simulink model "het_platoon_model"  (R2018b)
settings: Solver=ode1  StartTime=0.0  StopTime=simDrv.time_s(end)  FixedStep=sim_t_step  RelTol=1e-3
values from neighbouring files (symbols this model uses):
  sim_t_step = 0.01    [startHetPlatoonModel.m]
undefined symbols (not defined in the file or in its folder): adj_motEffMap, CTModel, DiscIntNeverNeededParam, LT, motSpdVec, motTrqVec, msk_mot_cont_trq, msk_mot_num, msk_mot_spd_bpt, MT, N_OptResults, simDrv, SPHETModel, TT
libraries: platooning_custom_blocks x24, simulink x7, dspstat3 x1, custom_func x1
(part 1 of 3)
PauseFcn:
  | runOptSPHET
settings Model: Creator=amankalia  LastModifiedBy=Aman-Home

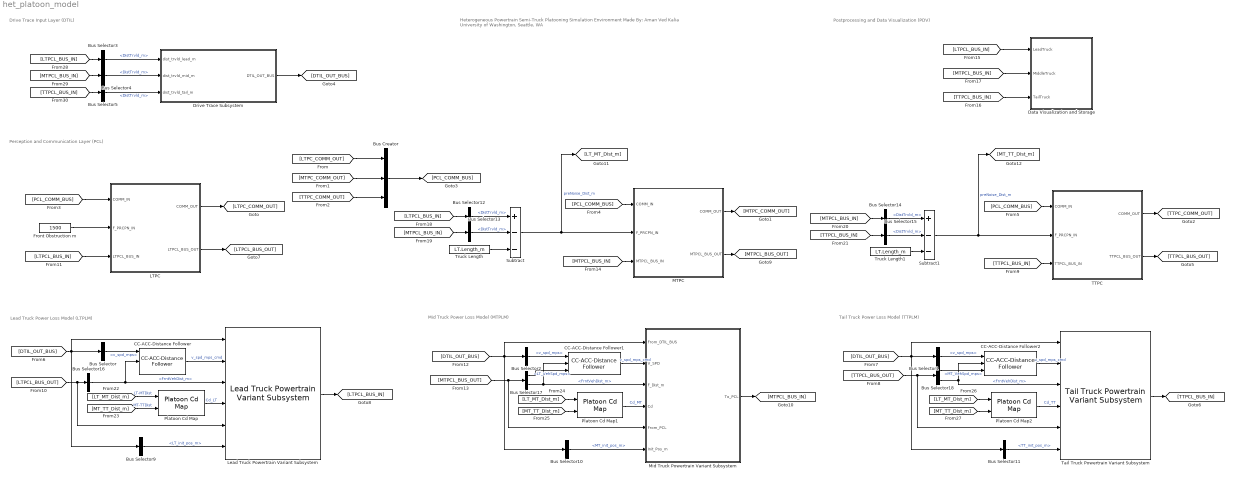
== system het_platoon_model ==
  note: Heterogeneous Powertrain Semi-Truck
      | Platooning Simulation Environment
      |
      | Made By: Aman Ved Kalia
      | University of Washington, Seattle, WA
  note: Lead Truck Power Loss Model (LTPLM)
  note: Perception and Communication Layer (PCL)
  note: Drive Trace Input Layer (DTIL)
  note: Mid Truck Power Loss Model (MTPLM)
  note: Tail Truck Power Loss Model (TTPLM)
  note: Postprocessing and Data Visualization (PDV)
  Bus Creator : BusCreator  Inputs=3
  Bus Selector : BusSelector  OutputSignals=v_spd_mps
  Bus Selector1 : BusSelector  OutputSignals=v_spd_mps
  Bus Selector10 : BusSelector  OutputSignals=MT_init_pos_m
  Bus Selector11 : BusSelector  OutputSignals=TT_init_pos_m
  Bus Selector{3..5,12..15} (7 alike) : BusSelector  OutputSignals=State_BUS.DistTrvld_m
  Bus Selector16 : BusSelector  OutputSignals=FrntVehDist_m
  Bus Selector17 : BusSelector  OutputSignals=LT_VehSpd_mps,FrntVehDist_m
  Bus Selector18 : BusSelector  OutputSignals=MT_VehSpd_mps,FrntVehDist_m
  Bus Selector2 : BusSelector  OutputSignals=v_spd_mps
  Bus Selector9 : BusSelector  OutputSignals=LT_init_pos_m
  CC-ACC-Distance Follower : platooning_custom_blocks/CC-ACC-Distance Follower  msk_cc_mode=Disabled  msk_cc_setspd=25  msk_cc_time=100  msk_ACC_Kp=0.5  msk_ACC_Ki=0.01  msk_ACC_Kd=0  msk_ACC_setdist_init=70  msk_platoon_time=200  msk_ACC_setdist_final=15
  CC-ACC-Distance Follower1 : platooning_custom_blocks/CC-ACC-Distance Follower  msk_cc_mode=Disabled  msk_cc_setspd=28  msk_cc_time=100  msk_ACC_Kp=1  msk_ACC_Ki=0.05  msk_ACC_Kd=0.01  msk_ACC_setdist_init=60  msk_platoon_time=200  msk_ACC_setdist_final=40
  CC-ACC-Distance Follower2 : platooning_custom_blocks/CC-ACC-Distance Follower  msk_cc_mode=Disabled  msk_cc_setspd=28  msk_cc_time=100  msk_ACC_Kp=1  msk_ACC_Ki=0.05  msk_ACC_Kd=0.01  msk_ACC_setdist_init=60  msk_platoon_time=200  msk_ACC_setdist_final=40
  Data Visualization and Storage : Subsystem
  Drive Trace Subsystem : Subsystem
  Front Obstruction m : Constant  Value=1500
  LTPC : Subsystem
  Lead Truck Powertrain Variant Subsystem : platooning_custom_blocks/Lead Truck Powertrain Variant Subsystem  SystemSampleTime=-1
  MTPC : Subsystem
  Mid Truck Powertrain Variant Subsystem : Subsystem  AncestorBlock=platooning_custom_blocks/Mid Truck Powertrain Variant Subsystem  Variant=on
  Platoon Cd Map : platooning_custom_blocks/Platoon Cd Map  msk_platoon_type=Individual  pos=Lead  msk_platoon_cd_map=Cd_Map  msk_platoon_cd_map_t2=Cd_Map_T2  msk_d1_bpt=d_11  msk_d2_bpt=d_22  msk_cd_avg=0.52
  Platoon Cd Map1 : platooning_custom_blocks/Platoon Cd Map  msk_platoon_type=Individual  pos=Middle  msk_platoon_cd_map=Cd_Map  msk_platoon_cd_map_t2=Cd_Map_T2  msk_d1_bpt=d_11  msk_d2_bpt=d_22  msk_cd_avg=0.52
  Platoon Cd Map2 : platooning_custom_blocks/Platoon Cd Map  msk_platoon_type=Individual  pos=Tail  msk_platoon_cd_map=Cd_Map  msk_platoon_cd_map_t2=Cd_Map_T2  msk_d1_bpt=d_11  msk_d2_bpt=d_22  msk_cd_avg=0.52
  Subtract : Sum  Inputs=+--
  Subtract1 : Sum  Inputs=+--
  TTPC : Subsystem
  Tail Truck Powertrain Variant Subsystem : platooning_custom_blocks/Tail Truck Powertrain Variant Subsystem  SystemSampleTime=-1
  Truck Length : Constant  Value=LT.Length_m
  Truck Length1 : Constant  Value=LT.Length_m
  wires:
  Drive Trace Subsystem/1(DTIL_OUT_BUS) -> [DTIL_OUT_BUS]
  LTPC/1(COMM_OUT) -> [LTPC_COMM_OUT]
  MTPC/1(COMM_OUT) -> [MTPC_COMM_OUT]
  TTPC/1(COMM_OUT) -> [TTPC_COMM_OUT]
  [LTPC_COMM_OUT] -> Bus Creator/1
  [MTPC_COMM_OUT] -> Bus Creator/2
  [TTPC_COMM_OUT] -> Bus Creator/3
  Bus Creator/1 -> [PCL_COMM_BUS]
  Bus Selector16/1 -> Lead Truck Powertrain Variant Subsystem/3, CC-ACC-Distance Follower/2  "<FrntVehDist_m>"
  Bus Selector/1 -> CC-ACC-Distance Follower/1  "<v_spd_mps>"
  [DTIL_OUT_BUS] -> Bus Selector/1, Lead Truck Powertrain Variant Subsystem/1, Bus Selector9/1
  CC-ACC-Distance Follower/1 -> Lead Truck Powertrain Variant Subsystem/2  "v_spd_mps_cmd"
  Bus Selector18/2 -> Tail Truck Powertrain Variant Subsystem/3, CC-ACC-Distance Follower2/2  "<FrntVehDist_m>"
  [DTIL_OUT_BUS] -> Bus Selector11/1, Bus Selector1/1, Tail Truck Powertrain Variant Subsystem/1
  Bus Selector1/1 -> CC-ACC-Distance Follower2/1  "<v_spd_mps>"
  CC-ACC-Distance Follower2/1 -> Tail Truck Powertrain Variant Subsystem/2  "v_spd_mps_cmd"
  TTPC/2(TTPCL_BUS_OUT) -> [TTPCL_BUS_OUT]
  [TTPCL_BUS_OUT] -> Tail Truck Powertrain Variant Subsystem/5, Bus Selector18/1
  Tail Truck Powertrain Variant Subsystem/1 -> [TTPCL_BUS_IN]
  [TTPCL_BUS_IN] -> TTPC/3(TTPCL_BUS_IN)
  LTPC/2(LTPCL_BUS_OUT) -> [LTPCL_BUS_OUT]
  [LTPCL_BUS_OUT] -> Bus Selector16/1, Lead Truck Powertrain Variant Subsystem/5
  Lead Truck Powertrain Variant Subsystem/1 -> [LTPCL_BUS_IN]
  [LTPCL_BUS_IN] -> LTPC/3(LTPCL_BUS_IN)
  [DTIL_OUT_BUS] -> Bus Selector10/1, Mid Truck Powertrain Variant Subsystem/1(From_DTIL_BUS), Bus Selector2/1
  CC-ACC-Distance Follower1/1 -> Mid Truck Powertrain Variant Subsystem/2(V_SPD)  "v_spd_mps_cmd"
  Bus Selector17/2 -> Mid Truck Powertrain Variant Subsystem/3(F_Dist_m), CC-ACC-Distance Follower1/2  "<FrntVehDist_m>"
  [MTPCL_BUS_OUT] -> Mid Truck Powertrain Variant Subsystem/5(From_PCL), Bus Selector17/1
  Bus Selector2/1 -> CC-ACC-Distance Follower1/1  "<v_spd_mps>"
  Mid Truck Powertrain Variant Subsystem/1(To_PCL) -> [MTPCL_BUS_IN]
  MTPC/2(MTPCL_BUS_OUT) -> [MTPCL_BUS_OUT]
  [MTPCL_BUS_IN] -> MTPC/3(MTPCL_BUS_IN)
  [PCL_COMM_BUS] -> LTPC/1(COMM_IN)
  [PCL_COMM_BUS] -> MTPC/1(COMM_IN)
  [PCL_COMM_BUS] -> TTPC/1(COMM_IN)
  Bus Selector9/1 -> Lead Truck Powertrain Variant Subsystem/6  "<LT_init_pos_m>"
  Bus Selector10/1 -> Mid Truck Powertrain Variant Subsystem/6(Init_Pos_m)  "<MT_init_pos_m>"
  Bus Selector11/1 -> Tail Truck Powertrain Variant Subsystem/6  "<TT_init_pos_m>"
  [LTPCL_BUS_IN] -> Bus Selector12/1
  [MTPCL_BUS_IN] -> Bus Selector13/1
  Bus Selector12/1 -> Subtract/1  "<DistTrvld_m>"
  Bus Selector13/1 -> Subtract/2  "<DistTrvld_m>"
  Truck Length/1 -> Subtract/3
  Truck Length1/1 -> Subtract1/3
  Bus Selector14/1 -> Subtract1/1  "<DistTrvld_m>"
  Bus Selector15/1 -> Subtract1/2  "<DistTrvld_m>"
  [MTPCL_BUS_IN] -> Bus Selector14/1
  [TTPCL_BUS_IN] -> Bus Selector15/1
  Front Obstruction m/1 -> LTPC/2(F_PRCPN_IN)
  Bus Selector17/1 -> CC-ACC-Distance Follower1/3  "<LT_VehSpd_mps>"
  Bus Selector18/1 -> CC-ACC-Distance Follower2/3  "<MT_VehSpd_mps>"
  Platoon Cd Map/1 -> Lead Truck Powertrain Variant Subsystem/4  "Cd_LT"
  [LT_MT_Dist_m] -> Platoon Cd Map/1  "LT-MTDist"
  [MT_TT_Dist_m] -> Platoon Cd Map/2  "MT-TTDist"
  [MT_TT_Dist_m] -> Platoon Cd Map1/2
  [LT_MT_Dist_m] -> Platoon Cd Map1/1
  Platoon Cd Map1/1 -> Mid Truck Powertrain Variant Subsystem/4(Cd)  "Cd_MT"
  [MT_TT_Dist_m] -> Platoon Cd Map2/2
  [LT_MT_Dist_m] -> Platoon Cd Map2/1
  Platoon Cd Map2/1 -> Tail Truck Powertrain Variant Subsystem/4  "Cd_TT"
  Subtract1/1 -> [MT_TT_Dist_m], TTPC/2(F_PRCPN_IN)  "preNoise_Dist_m"
  Subtract/1 -> [LT_MT_Dist_m], MTPC/2(F_PRCPN_IN)  "preNoise_Dist_m"
  [LTPCL_BUS_IN] -> Data Visualization and Storage/1(LeadTruck)
  [MTPCL_BUS_IN] -> Data Visualization and Storage/2(MiddleTruck)
  [TTPCL_BUS_IN] -> Data Visualization and Storage/3(TailTruck)
  [LTPCL_BUS_IN] -> Bus Selector3/1
  Bus Selector3/1 -> Drive Trace Subsystem/1(dist_trvld_lead_m)  "<DistTrvld_m>"
  [MTPCL_BUS_IN] -> Bus Selector4/1
  Bus Selector4/1 -> Drive Trace Subsystem/2(dist_trvld_mid_m)  "<DistTrvld_m>"
  [TTPCL_BUS_IN] -> Bus Selector5/1
  Bus Selector5/1 -> Drive Trace Subsystem/3(dist_trvld_tail_m)  "<DistTrvld_m>"

== system het_platoon_model/Data Visualization and Storage ==
  LeadTruck : Inport
  MiddleTruck : Inport  Port=2
  TailTruck : Inport  Port=3
  Bus Creator : BusCreator  Inputs=3
  Bus Creator1 : BusCreator  Inputs=3
  Bus Creator2 : BusCreator  Inputs=3
  Bus Selector3 : BusSelector  OutputSignals=EC_BUS,FC_BUS,State_BUS
  Bus Selector5 : BusSelector  OutputSignals=EC_BUS,State_BUS,FC_BUS
  Bus Selector7 : BusSelector  OutputSignals=EC_BUS,FC_BUS,State_BUS
  Scope{,1..7} (8 alike) : Scope
  To Workspace : ToWorkspace  VariableName=TT_SimData  SaveFormat=Timeseries  SampleTime=-1
  To Workspace1 : ToWorkspace  VariableName=LT_SimData  SaveFormat=Timeseries  SampleTime=-1
  To Workspace2 : ToWorkspace  VariableName=MT_SimData  SaveFormat=Timeseries  SampleTime=-1
  wires:
  Bus Selector3/2 -> Bus Creator1/2, Scope1/1  "<FC_BUS>"
  Bus Selector7/3 -> Scope7/1, Bus Creator2/3  "<State_BUS>"
  Bus Selector5/1 -> Bus Creator/1, Scope3/1  "<EC_BUS>"
  Bus Selector7/1 -> Bus Creator2/1, Scope5/1  "<EC_BUS>"
  Bus Selector3/3 -> Scope2/1, Bus Creator1/3  "<State_BUS>"
  TailTruck/1 -> Bus Selector5/1
  Bus Selector5/2 -> Scope4/1, Bus Creator/2  "<State_BUS>"
  Bus Selector7/2 -> Bus Creator2/2, Scope6/1  "<FC_BUS>"
  Bus Selector3/1 -> Bus Creator1/1, Scope/1  "<EC_BUS>"
  LeadTruck/1 -> Bus Selector3/1
  MiddleTruck/1 -> Bus Selector7/1
  Bus Creator/1 -> To Workspace/1
  Bus Creator1/1 -> To Workspace1/1
  Bus Creator2/1 -> To Workspace2/1
  Bus Selector5/3 -> Bus Creator/3  "<FC_BUS>"

== system het_platoon_model/Drive Trace Subsystem ==
  note: simDrv.dist_mi * 1609.34
  note: simDrv.rand_spd_mph * 0.44704
  dist_trvld_lead_m : Inport
  dist_trvld_mid_m : Inport  Port=2
  dist_trvld_tail_m : Inport  Port=3
  Bus Creator : BusCreator  Inputs=8
  Clock : Clock
  Constant : Constant  Value=LT.Init_Pos_m
  Constant1 : Constant  Value=MT.Init_Pos_m
  Constant2 : Constant  Value=TT.Init_Pos_m
  Cycle Distance : Constant  Commented=on  Value=simDrv.dist_mi(end) * 1609.34
  Distance vs Grade LUT1 : Lookup_n-D  NumberOfTableDimensions=1  BreakpointsForDimension1=simDrv.dist_m(2:6)  Table=simDrv.grade_pct(2:6)  ExtrapMethod=Clip  UseLastTableValue=on  InternalRulePriority=Speed  RndMeth=Simplest  InputSameDT=on
  Distance vs Grade LUT2 : Lookup_n-D  NumberOfTableDimensions=1  BreakpointsForDimension1=simDrv.dist_m(2:6)  Table=simDrv.grade_pct(2:6)  ExtrapMethod=Clip  UseLastTableValue=on  InternalRulePriority=Speed  RndMeth=Simplest  InputSameDT=on
  Distance vs Grade LUT3 : Lookup_n-D  NumberOfTableDimensions=1  BreakpointsForDimension1=simDrv.dist_m(2:6)  Table=simDrv.grade_pct(2:6)  ExtrapMethod=Clip  UseLastTableValue=on  InternalRulePriority=Speed  RndMeth=Simplest  InputSameDT=on
  GreaterThan : RelationalOperator  Commented=on  OutDataTypeStr=boolean  RndMeth=Simplest
  GreaterThan1 : RelationalOperator  Commented=on  OutDataTypeStr=boolean  RndMeth=Simplest
  GreaterThan2 : RelationalOperator  Commented=on  OutDataTypeStr=boolean  RndMeth=Simplest
  Logical Operator : Logic  Commented=on  Inputs=3  AllPortsSameDT=off  OutDataTypeStr=boolean
  Speed vs Time LUT : Lookup_n-D  NumberOfTableDimensions=1  BreakpointsForDimension1=simDrv.time_s  Table=simDrv.spd_mps  ExtrapMethod=Clip  UseLastTableValue=on  InternalRulePriority=Speed  RndMeth=Simplest  InputSameDT=on
  Stop Simulation : Stop  Commented=on
  DTIL_OUT_BUS : Outport
  wires:
  dist_trvld_lead_m/1 -> GreaterThan/1, Distance vs Grade LUT1/1
  Bus Creator/1 -> DTIL_OUT_BUS/1  "DTIL_OUT_BUS"
  Distance vs Grade LUT1/1 -> Bus Creator/3  "lead_grade_pct"
  Speed vs Time LUT/1 -> Bus Creator/2  "v_spd_mps"
  Clock/1 -> Bus Creator/1, Speed vs Time LUT/1  "clock"
  dist_trvld_mid_m/1 -> GreaterThan1/1, Distance vs Grade LUT2/1
  dist_trvld_tail_m/1 -> GreaterThan2/1, Distance vs Grade LUT3/1
  Distance vs Grade LUT2/1 -> Bus Creator/4  "mid_grade_pct"
  Distance vs Grade LUT3/1 -> Bus Creator/5  "tail_grade_pct"
  Constant/1 -> Bus Creator/6  "LT_init_pos_m"
  Constant1/1 -> Bus Creator/7  "MT_init_pos_m"
  Constant2/1 -> Bus Creator/8  "TT_init_pos_m"
  Cycle Distance/1 -> GreaterThan/2, GreaterThan1/2, GreaterThan2/2
  GreaterThan1/1 -> Logical Operator/2
  GreaterThan/1 -> Logical Operator/1
  GreaterThan2/1 -> Logical Operator/3
  Logical Operator/1 -> Stop Simulation/1

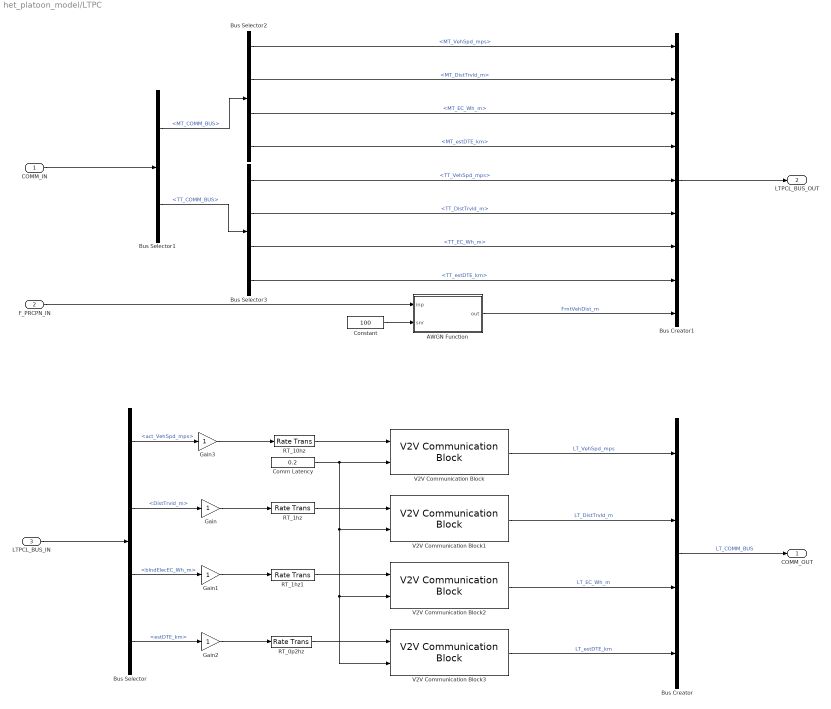
== system het_platoon_model/LTPC ==
  COMM_IN : Inport
  F_PRCPN_IN : Inport  Port=2
  LTPCL_BUS_IN : Inport  Port=3
  AWGN Function : MATLAB Function  TreatAsAtomicUnit=on
  Bus Creator : BusCreator  Inputs=4
  Bus Creator1 : BusCreator  Inputs=9
  Bus Selector : BusSelector  OutputSignals=State_BUS.act_VehSpd_mps,State_BUS.DistTrvld_m,EC_BUS.blndElecEC_Wh_m,State_BUS.estDTE_km
  Bus Selector1 : BusSelector  OutputSignals=MT_COMM_BUS,TT_COMM_BUS
  Bus Selector2 : BusSelector  OutputSignals=MT_VehSpd_mps,MT_DistTrvld_m,MT_EC_Wh_m,MT_estDTE_km
  Bus Selector3 : BusSelector  OutputSignals=TT_VehSpd_mps,TT_DistTrvld_m,TT_EC_Wh_m,TT_estDTE_km
  Comm Latency : Constant  Value=0.2
  Constant : Constant  Value=100
  Gain{,1..3} (4 alike) : Gain
  RT_0p2hz : RateTransition  OutPortSampleTime=1
  RT_10hz : RateTransition  OutPortSampleTime=0.1
  RT_1hz : RateTransition  OutPortSampleTime=1
  RT_1hz1 : RateTransition  OutPortSampleTime=1
  V2V Communication Block{,1..3} (4 alike) : platooning_custom_blocks/V2V Communication Block  msk_t_step_s=sim_t_step  msk_snr_value=100
  COMM_OUT : Outport
  LTPCL_BUS_OUT : Outport  Port=2
  wires:
  Bus Creator/1 -> COMM_OUT/1  "LT_COMM_BUS"
  Bus Creator1/1 -> LTPCL_BUS_OUT/1
  COMM_IN/1 -> Bus Selector1/1
  F_PRCPN_IN/1 -> AWGN Function/1(inp)
  LTPCL_BUS_IN/1 -> Bus Selector/1
  Bus Selector/2 -> Gain/1  "<DistTrvld_m>"
  Bus Selector/3 -> Gain1/1  "<blndElecEC_Wh_m>"
  Gain/1 -> RT_1hz/1
  Gain1/1 -> RT_1hz1/1
  Bus Selector/4 -> Gain2/1  "<estDTE_km>"
  Gain2/1 -> RT_0p2hz/1
  Constant/1 -> AWGN Function/2(snr)
  AWGN Function/1(out) -> Bus Creator1/9  "FrntVehDist_m"
  Bus Selector/1 -> Gain3/1  "<act_VehSpd_mps>"
  Gain3/1 -> RT_10hz/1
  RT_10hz/1 -> V2V Communication Block/1
  RT_1hz/1 -> V2V Communication Block1/1
  RT_1hz1/1 -> V2V Communication Block2/1
  RT_0p2hz/1 -> V2V Communication Block3/1
  V2V Communication Block3/1 -> Bus Creator/4  "LT_estDTE_km"
  V2V Communication Block2/1 -> Bus Creator/3  "LT_EC_Wh_m"
  V2V Communication Block1/1 -> Bus Creator/2  "LT_DistTrvld_m"
  V2V Communication Block/1 -> Bus Creator/1  "LT_VehSpd_mps"
  Comm Latency/1 -> V2V Communication Block3/2, V2V Communication Block2/2, V2V Communication Block1/2, V2V Communication Block/2
  Bus Selector1/1 -> Bus Selector2/1  "<MT_COMM_BUS>"
  Bus Selector1/2 -> Bus Selector3/1  "<TT_COMM_BUS>"
  Bus Selector3/4 -> Bus Creator1/8  "<TT_estDTE_km>"
  Bus Selector3/3 -> Bus Creator1/7  "<TT_EC_Wh_m>"
  Bus Selector3/2 -> Bus Creator1/6  "<TT_DistTrvld_m>"
  Bus Selector3/1 -> Bus Creator1/5  "<TT_VehSpd_mps>"
  Bus Selector2/4 -> Bus Creator1/4  "<MT_estDTE_km>"
  Bus Selector2/3 -> Bus Creator1/3  "<MT_EC_Wh_m>"
  Bus Selector2/2 -> Bus Creator1/2  "<MT_DistTrvld_m>"
  Bus Selector2/1 -> Bus Creator1/1  "<MT_VehSpd_mps>"

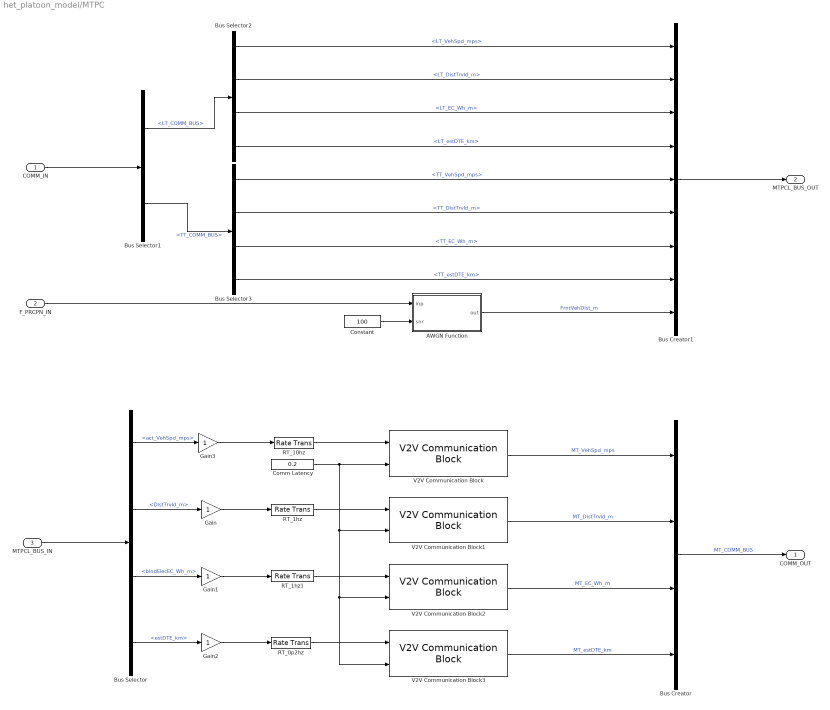
== system het_platoon_model/MTPC ==
  COMM_IN : Inport
  F_PRCPN_IN : Inport  Port=2
  MTPCL_BUS_IN : Inport  Port=3
  AWGN Function : MATLAB Function  TreatAsAtomicUnit=on
  Bus Creator : BusCreator  Inputs=4
  Bus Creator1 : BusCreator  Inputs=9
  Bus Selector : BusSelector  OutputSignals=State_BUS.act_VehSpd_mps,State_BUS.DistTrvld_m,EC_BUS.blndElecEC_Wh_m,State_BUS.estDTE_km
  Bus Selector1 : BusSelector  OutputSignals=LT_COMM_BUS,TT_COMM_BUS
  Bus Selector2 : BusSelector  OutputSignals=LT_VehSpd_mps,LT_DistTrvld_m,LT_EC_Wh_m,LT_estDTE_km
  Bus Selector3 : BusSelector  OutputSignals=TT_VehSpd_mps,TT_DistTrvld_m,TT_EC_Wh_m,TT_estDTE_km
  Comm Latency : Constant  Value=0.2
  Constant : Constant  Value=100
  Gain{,1..3} (4 alike) : Gain
  RT_0p2hz : RateTransition  OutPortSampleTime=1
  RT_10hz : RateTransition  OutPortSampleTime=0.1
  RT_1hz : RateTransition  OutPortSampleTime=1
  RT_1hz1 : RateTransition  OutPortSampleTime=1
  V2V Communication Block{,1..3} (4 alike) : platooning_custom_blocks/V2V Communication Block  msk_t_step_s=sim_t_step  msk_snr_value=100
  COMM_OUT : Outport
  MTPCL_BUS_OUT : Outport  Port=2
  wires:
  Bus Creator/1 -> COMM_OUT/1  "MT_COMM_BUS"
  Bus Creator1/1 -> MTPCL_BUS_OUT/1
  COMM_IN/1 -> Bus Selector1/1
  F_PRCPN_IN/1 -> AWGN Function/1(inp)
  MTPCL_BUS_IN/1 -> Bus Selector/1
  Bus Selector/2 -> Gain/1  "<DistTrvld_m>"
  Bus Selector/3 -> Gain1/1  "<blndElecEC_Wh_m>"
  Gain/1 -> RT_1hz/1
  Gain1/1 -> RT_1hz1/1
  Bus Selector/4 -> Gain2/1  "<estDTE_km>"
  Gain2/1 -> RT_0p2hz/1
  Constant/1 -> AWGN Function/2(snr)
  AWGN Function/1(out) -> Bus Creator1/9  "FrntVehDist_m"
  Bus Selector/1 -> Gain3/1  "<act_VehSpd_mps>"
  Gain3/1 -> RT_10hz/1
  RT_10hz/1 -> V2V Communication Block/1
  RT_1hz/1 -> V2V Communication Block1/1
  RT_1hz1/1 -> V2V Communication Block2/1
  RT_0p2hz/1 -> V2V Communication Block3/1
  V2V Communication Block3/1 -> Bus Creator/4  "MT_estDTE_km"
  V2V Communication Block2/1 -> Bus Creator/3  "MT_EC_Wh_m"
  V2V Communication Block1/1 -> Bus Creator/2  "MT_DistTrvld_m"
  V2V Communication Block/1 -> Bus Creator/1  "MT_VehSpd_mps"
  Comm Latency/1 -> V2V Communication Block3/2, V2V Communication Block2/2, V2V Communication Block1/2, V2V Communication Block/2
  Bus Selector3/3 -> Bus Creator1/7  "<TT_EC_Wh_m>"
  Bus Selector3/1 -> Bus Creator1/5  "<TT_VehSpd_mps>"
  Bus Selector2/2 -> Bus Creator1/2  "<LT_DistTrvld_m>"
  Bus Selector3/2 -> Bus Creator1/6  "<TT_DistTrvld_m>"
  Bus Selector2/4 -> Bus Creator1/4  "<LT_estDTE_km>"
  Bus Selector3/4 -> Bus Creator1/8  "<TT_estDTE_km>"
  Bus Selector2/1 -> Bus Creator1/1  "<LT_VehSpd_mps>"
  Bus Selector1/1 -> Bus Selector2/1  "<LT_COMM_BUS>"
  Bus Selector2/3 -> Bus Creator1/3  "<LT_EC_Wh_m>"
  Bus Selector1/2 -> Bus Selector3/1  "<TT_COMM_BUS>"

== system het_platoon_model/Mid Truck Powertrain Variant Subsystem ==
  note: 1) Add Subsystem or Model blocks as valid variant choices.
      | 2) You cannot connect blocks at this level. At simulation, connectivity is automatically
      | determined, based on the active variant and port name matching.
  From_DTIL_BUS : Inport
  V_SPD : Inport  Port=2
  F_Dist_m : Inport  Port=3
  Cd : Inport  Port=4
  From_PCL : Inport  Port=5
  Init_Pos_m : Inport  Port=6
  Battery Electric Truck : platooning_custom_blocks/Battery Electric Truck  SystemSampleTime=-1  VariantControl=MT.Type == 3
  Conventional Truck : platooning_custom_blocks/Conventional Truck  SystemSampleTime=-1  VariantControl=MT.Type == 1
  Series Parallel Hybrid Electric Truck : Subsystem  AncestorBlock=platooning_custom_blocks/Series Parallel Hybrid Electric Truck  VariantControl=MT.Type == 2
  To_PCL : Outport

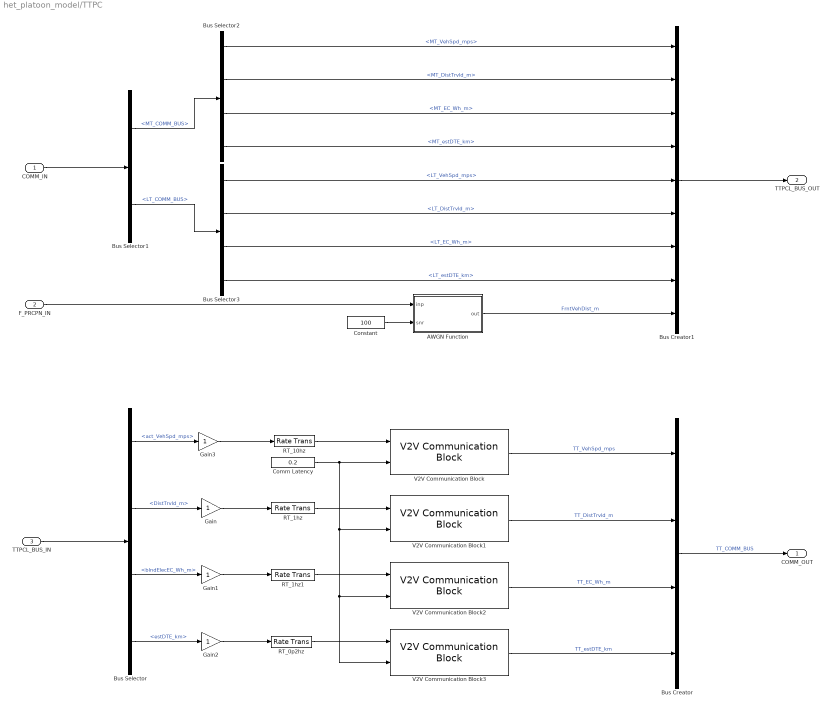
== system het_platoon_model/TTPC ==
  COMM_IN : Inport
  F_PRCPN_IN : Inport  Port=2
  TTPCL_BUS_IN : Inport  Port=3
  AWGN Function : MATLAB Function  TreatAsAtomicUnit=on
  Bus Creator : BusCreator  Inputs=4
  Bus Creator1 : BusCreator  Inputs=9
  Bus Selector : BusSelector  OutputSignals=State_BUS.act_VehSpd_mps,State_BUS.DistTrvld_m,EC_BUS.blndElecEC_Wh_m,State_BUS.estDTE_km
  Bus Selector1 : BusSelector  OutputSignals=MT_COMM_BUS,LT_COMM_BUS
  Bus Selector2 : BusSelector  OutputSignals=MT_VehSpd_mps,MT_DistTrvld_m,MT_EC_Wh_m,MT_estDTE_km
  Bus Selector3 : BusSelector  OutputSignals=LT_VehSpd_mps,LT_DistTrvld_m,LT_EC_Wh_m,LT_estDTE_km
  Comm Latency : Constant  Value=0.2
  Constant : Constant  Value=100
  Gain{,1..3} (4 alike) : Gain
  RT_0p2hz : RateTransition  OutPortSampleTime=1
  RT_10hz : RateTransition  OutPortSampleTime=0.1
  RT_1hz : RateTransition  OutPortSampleTime=1
  RT_1hz1 : RateTransition  OutPortSampleTime=1
  V2V Communication Block{,1..3} (4 alike) : platooning_custom_blocks/V2V Communication Block  msk_t_step_s=sim_t_step  msk_snr_value=100
  COMM_OUT : Outport
  TTPCL_BUS_OUT : Outport  Port=2
  wires:
  Bus Creator/1 -> COMM_OUT/1  "TT_COMM_BUS"
  Bus Creator1/1 -> TTPCL_BUS_OUT/1
  COMM_IN/1 -> Bus Selector1/1
  F_PRCPN_IN/1 -> AWGN Function/1(inp)
  TTPCL_BUS_IN/1 -> Bus Selector/1
  Bus Selector/2 -> Gain/1  "<DistTrvld_m>"
  Bus Selector/3 -> Gain1/1  "<blndElecEC_Wh_m>"
  Gain/1 -> RT_1hz/1
  Gain1/1 -> RT_1hz1/1
  Bus Selector/4 -> Gain2/1  "<estDTE_km>"
  Gain2/1 -> RT_0p2hz/1
  Constant/1 -> AWGN Function/2(snr)
  AWGN Function/1(out) -> Bus Creator1/9  "FrntVehDist_m"
  Bus Selector/1 -> Gain3/1  "<act_VehSpd_mps>"
  Gain3/1 -> RT_10hz/1
  RT_10hz/1 -> V2V Communication Block/1
  RT_1hz/1 -> V2V Communication Block1/1
  RT_1hz1/1 -> V2V Communication Block2/1
  RT_0p2hz/1 -> V2V Communication Block3/1
  V2V Communication Block3/1 -> Bus Creator/4  "TT_estDTE_km"
  V2V Communication Block2/1 -> Bus Creator/3  "TT_EC_Wh_m"
  V2V Communication Block1/1 -> Bus Creator/2  "TT_DistTrvld_m"
  V2V Communication Block/1 -> Bus Creator/1  "TT_VehSpd_mps"
  Comm Latency/1 -> V2V Communication Block3/2, V2V Communication Block2/2, V2V Communication Block1/2, V2V Communication Block/2
  Bus Selector3/3 -> Bus Creator1/7  "<LT_EC_Wh_m>"
  Bus Selector3/1 -> Bus Creator1/5  "<LT_VehSpd_mps>"
  Bus Selector2/2 -> Bus Creator1/2  "<MT_DistTrvld_m>"
  Bus Selector3/2 -> Bus Creator1/6  "<LT_DistTrvld_m>"
  Bus Selector2/4 -> Bus Creator1/4  "<MT_estDTE_km>"
  Bus Selector3/4 -> Bus Creator1/8  "<LT_estDTE_km>"
  Bus Selector2/1 -> Bus Creator1/1  "<MT_VehSpd_mps>"
  Bus Selector1/1 -> Bus Selector2/1  "<MT_COMM_BUS>"
  Bus Selector2/3 -> Bus Creator1/3  "<MT_EC_Wh_m>"
  Bus Selector1/2 -> Bus Selector3/1  "<LT_COMM_BUS>"

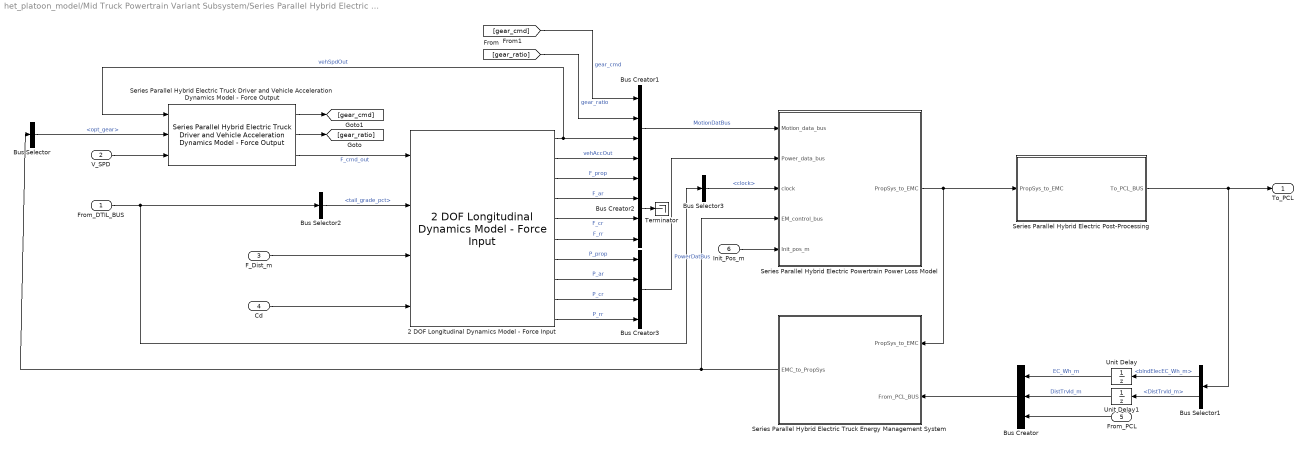
== system het_platoon_model/Mid Truck Powertrain Variant Subsystem/Series Parallel Hybrid Electric Truck ==
  From_DTIL_BUS : Inport
  V_SPD : Inport  Port=2
  F_Dist_m : Inport  Port=3
  Cd : Inport  Port=4
  From_PCL : Inport  Port=5
  Init_Pos_m : Inport  Port=6
  2 DOF Longitudinal Dynamics Model - Force Input : platooning_custom_blocks/2 DOF Longitudinal Dynamics Model - Force Input  msk_mass=SPHETModel.veh_mass_kg  msk_Af=SPHETModel.Af_m2  msk_Cd=SPHETModel.Cd_avg * ones([3 1])  msk_Cd_bpt=[5;10;15]  msk_r_tire=SPHETModel.ld_tire_rad_m  msk_v_init=init_veh_spd_mps  msk_roadType=Smooth Concrete  msk_rho_air=1.227  msk_tstep=sim_t_step
  Bus Creator : BusCreator  Inputs=3
  Bus Creator1 : BusCreator  Inputs=4
  Bus Creator2 : BusCreator  Inputs=4
  Bus Creator3 : BusCreator  Inputs=4
  Bus Selector : BusSelector  OutputSignals=opt_gear
  Bus Selector1 : BusSelector  OutputSignals=EC_BUS.blndElecEC_Wh_m,State_BUS.DistTrvld_m
  Bus Selector2 : BusSelector  OutputSignals=tail_grade_pct
  Bus Selector3 : BusSelector  OutputSignals=clock
  Series Parallel Hybrid Electric Post-Processing : Subsystem  mask{msk_cell_Q_Ah=SPHETModel.Q_cell_max_Ah, msk_cell_Vnom=SPHETModel.V_cell_nom, msk_batt_Ns=SPHETModel.Ns, msk_batt_Np=SPHETModel.Np, msk_batt_Nmod=SPHETModel.Nmod, msk_batt_soc_init=0.8, msk_fuel_init_liters=SPHETModel.fuelTankCap_L, msk_fuel_rho_kgpl=SPHETModel.fuelrho_kgpl, msk_fuel_lhv_kwhpkg=SPHETModel.fuelLHV_kwhpkg, msk_distwin=1000}
      mask prompts: msk_cell_Q_Ah "Battery cell capacity, Q [Ah]:"; msk_cell_Vnom "Battery cell nominal voltage, Vnom [V]:"; msk_batt_Ns "Number of cells in series, Ns [-]:"; msk_batt_Np "Number of cells in parallel, Np [-]:"; msk_batt_Nmod "Number of modules, Nmod [-]:"; msk_batt_soc_init "Battery initial SOC, SOCinit/100 :"; msk_fuel_init_liters "Initial fuel capacity [US gallons]:"; msk_fuel_rho_kgpl "Fuel density [kg/L]:"; msk_fuel_lhv_kwhpkg "Fuel LHV [kWh/kg]:"; msk_distwin "Short term averaging, distance window [m]:"
      mask DialogControl DescGroupVar Prompt: Post-Processing Block - Battery Electric Vehicle
      mask DialogControl DescTextVar Prompt: This block computes overall energy consumption and distance-to-empty for a battery electric vehicle.
      mask DialogControl ParameterGroupVar Prompt: Battery Parameters
      mask DialogControl Container3 Prompt: Fuel Parameters
      mask DialogControl Container4 Prompt: Averaging Parameters
  Series Parallel Hybrid Electric Powertrain Power Loss Model : Subsystem  mask{msk_eng_pk_trq_vec=SPHETModel.peak_eng_trq_map, msk_eng_pk_mtr_trq=SPHETModel.mtr_eng_trq_map, msk_eng_trq_spd_bpt=SPHETModel.peak_eng_trq_spd_bpt, msk_eng_fuel_map=SPHETModel.eng_fuel_map, msk_eng_trq_bpt=SPHETModel.eng_map_trq_bpt, msk_eng_spd_bpt=SPHETModel.eng_map_spd_bpt, msk_fuel_init_liters=SPHETModel.fuelTankCap_L, msk_rho_fuel_kgpL=SPHETModel.fuelrho_kgpl, msk_gen_ctl_Kp=0.1, msk_gen_ctl_Ki=0.001, msk_gen_mtr_cont_trq=SPHETModel.cont_gen_mtr_trq_map, msk_gen_mtr_eff_map=SPHETModel.gen_mtr_eff_map, msk_gen_mtr_trqbpt=SPHETModel.gen_mtr_trqbpt, msk_gen_mtr_spdbpt=SPHETModel.gen_mtr_spdbpt, msk_mot_eff=SPHETModel.mtr_eff, msk_gear_ratio_vec=SPHETModel.gear_ratios, msk_gear_eff_vec=SPHETModel.gear_eff, msk_fd_ratio=SPHETModel.fd_ratio, msk_drv_eff=0.98, msk_plnt_m_r_ratio=SPHETModel.mg_ratio_mot_out, msk_plnt_c_r_ratio=SPHETModel.mg_ratio_eng_out, msk_plnt_s_r_ratio=1/SPHETModel.mg_ratio_out_gen, msk_plnt_c_s_ratio=SPHETModel.mg_ratio_eng_gen, msk_plnt_gear_eff=SPHETModel.plnt_gear_eff, msk_tire_radius_m=SPHETModel.ld_tire_rad_m, msk_cell_Q_Ah=SPHETModel.Q_cell_max_Ah, msk_cell_Vnom=SPHETModel.V_cell_nom, msk_batt_Ns=SPHETModel.Ns, msk_batt_Np=SPHETModel.Np, msk_batt_Nmod=SPHETModel.Nmod, msk_batt_soc_init=0.8, msk_dchglim10s=SPHETModel.DchgCurrLim_10sAvg_A, msk_cellTempbpt=SPHETModel.cellTempbpt_C, msk_soc_bpt=SPHETModel.socbpt, msk_batt_R0=SPHETModel.batt_R0, msk_batt_R1=SPHETModel.batt_R1, msk_batt_R2=SPHETModel.batt_R2, msk_batt_C1=SPHETModel.batt_C1, msk_batt_C2=SPHETModel.batt_C2, msk_batt_soc_bpt=SPHETModel.batt_socbpt, msk_P_aux_mech_load=SPHETModel.P_aux_mech, msk_P_aux_elec_load=SPHETModel.P_aux_elec, msk_P_aux_load_frac=SPHETModel.P_aux_load_frac, msk_snr_P_aux=25, msk_t_step=sim_t_step}
      mask prompts: msk_eng_pk_trq_vec "Engine peak torque vector, propulsion [] :"; msk_eng_pk_mtr_trq "Engine peak torque vector, motoring [] :"; msk_eng_trq_spd_bpt "Engine torque speed breakpoint [] :"; msk_eng_fuel_map "Engine fuel map, g/s [] :"; msk_eng_trq_bpt "Engine torque breakpoint []:"; msk_eng_spd_bpt "Engine speed breakpoint []:"; msk_fuel_init_liters "Initial fuel capacity [Liters] :"; msk_rho_fuel_kgpL "Fuel density [kg/L] :"; msk_gen_ctl_Kp "Generator load control, Proportional Gain :"; msk_gen_ctl_Ki "Generator load control, Integrator Gain :"; msk_gen_mtr_cont_trq "Generator continuous torque vector [] :"; msk_gen_mtr_eff_map "Generator motor efficiency map [] :"; msk_gen_mtr_trqbpt "Generator motor torque breakpoint [] :"; msk_gen_mtr_spdbpt "Generator speed breakpoint [] :"; msk_mot_eff "Motor efficiency/100 [-]:"; msk_gear_ratio_vec "Gear ratio vector []:"; msk_gear_eff_vec "Gear efficiency vector []:"; msk_fd_ratio "Final drive ratio :"; msk_drv_eff "Driveline efficiency :"; msk_plnt_m_r_ratio "Motor to Output ratio (M to R) :"; msk_plnt_c_r_ratio "Engine to Output ratio (C to R) :"; msk_plnt_s_r_ratio "Generator to Output ratio (S to R) :"; msk_plnt_c_s_ratio "Engine to Generator ratio (C to S) :"; msk_plnt_gear_eff "Planetary gearbox efficiency :"; msk_tire_radius_m "Loaded tire radius [m]:"; msk_cell_Q_Ah "Battery cell capacity, Q [Ah]:"; msk_cell_Vnom "Battery cell nominal voltage, Vnom [V]:"; msk_batt_Ns "Number of cells in series, Ns [-]:"; msk_batt_Np "Number of cells in parallel, Np [-]:"; msk_batt_Nmod "Number of battery modules, Nmod [-]:"; msk_batt_soc_init "Battery initial SOC [SOC/100]:"; msk_dchglim10s "Battery 10s Discharge Limit []:"; msk_cellTempbpt "Battery cell temperature breakpoint []:"; msk_soc_bpt "Battery SOC breakpoint []:"; msk_batt_R0 "Battery Resistance R0 LUT []:"; msk_batt_R1 "Battery Resistance R1 LUT []:"; msk_batt_R2 "Battery Resistance R2 LUT []:"; msk_batt_C1 "Battery Capacitance C1 LUT []:"; msk_batt_C2 "Battery Capacitance C2 LUT []:"; msk_batt_soc_bpt "Battery internal params SOC breakpoints []:"; msk_P_aux_mech_load "Auxiliary load power, mechanical [W]:"; msk_P_aux_elec_load "Auxiliary load power, electrical [W]:"; msk_P_aux_load_frac "Auxiliary load fraction [-]"; msk_snr_P_aux "Signal-to-Noise ratio [-]:"; msk_t_step "Simulation time step [s]:"
      mask DialogControl DescGroupVar Prompt: Battery Electric Powertrain Mode
      mask DialogControl DescTextVar Prompt: Parameter settings for systems and components in the Battery Electric Powertrain
      mask DialogControl Container7 Prompt: Drivetrain Parameters
      mask DialogControl Container12 Prompt: Engine Parameters
      mask DialogControl Container18 Prompt: Fuel Parameters
      mask DialogControl Container13 Prompt: Generator Parameters
      mask DialogControl Container9 Prompt: Motor Parameters
      mask DialogControl Container14 Prompt: Transmission Parameters
      mask DialogControl Container16 Prompt: P2 Hybrid Planetary Gearbox
      mask DialogControl Container15 Prompt: Vehicle Parameters
      mask DialogControl Container10 Prompt: Battery Parameters
      mask DialogControl Container4 Prompt: Internal Battery Parameters
      mask DialogControl Container11 Prompt: Auxiliary Load Parameters
      mask DialogControl Container17 Prompt: Simulation Parameters
  Series Parallel Hybrid Electric Truck Energy Management System : Subsystem  mask{msk_algoChoice=Standard SPHET Algo, msk_regen_pwr_vec=SPHETModel.mtr_regen_pwr_vec, msk_regen_spd_bpt=SPHETModel.mtr_regen_pwr_spdbpt, msk_DistVector=simDrv.dist_m, msk_OptHybMode=N_OptResults.HybModeGrp, msk_OptGenPwr=N_OptResults.optPgen_W, msk_OptMotPwr=N_OptResults.optPmot_W, msk_OptSOC=N_OptResults.optSOC_pct, msk_OptEC=N_OptResults.EC_Wh_m}
      mask prompts: msk_algoChoice "Energy Management Algorithm Choice"; msk_regen_pwr_vec "Motor regen power vector, watts []:"; msk_regen_spd_bpt "Motor regen power breakpoint - vehicle speed, mps []:"; msk_DistVector "Distance Vector:"; msk_OptHybMode "Optimal Hybrid Mode Vector:"; msk_OptGenPwr "Optimal Generator Power Vector:"; msk_OptMotPwr "Optimal Motor Power Vector:"; msk_OptSOC "Optimal SOC Vector:"; msk_OptEC "Optimal EC Vector:"
      mask init:
      | switch msk_algoChoice
      |     case 'DC-ARTDP Algo'
      |         msk_algoChoice = 1;
      |     case 'Standard SPHET Algo'
      |         msk_algoChoice = 2;
      | end
      mask TypeOptions msk_algoChoice: DC-ARTDP Algo | Standard SPHET Algo
      mask DialogControl DescGroupVar Prompt: Battery Electric Energy Management System
      mask DialogControl DescTextVar Prompt: Parameter settings for the Battery Electric Energy Management Systems
      mask DialogControl Container3 Prompt: DC-ARTDP Algorithm Parameters
  Series Parallel Hybrid Electric Truck Driver and Vehicle Acceleration Dynamics Model - Force Output : platooning_custom_blocks/Series Parallel Hybrid Electric Truck Driver and  Vehicle Acceleration Dynamics Model  - Force Output  msk_mass=SPHETModel.veh_mass_kg  msk_damp_acc=800  msk_damp_brk=0.1  msk_tire_radius=SPHETModel.ld_tire_rad_m  msk_brk_whl_num=18  msk_fd_ratio=SPHETModel.fd_ratio  msk_Kp=0.1  msk_Ki=0.001  msk_t_step=sim_t_step  msk_eng_pk_trq=SPHETModel.peak_eng_trq_map  msk_eng_spd_bpt=SPHETModel.peak_eng_trq_spd_bpt  msk_gear_ratio_vec=SPHETModel.gear_ratios  msk_gearInit=1  msk_gearShft_UL=[3, 5, 9, 13, 17, 21, 25, 29, 33, 45]  msk_gearShft_LL=[0, 2, 4, 8, 12, 16, 20, 24, 28, 32]  msk_plnt_c_r_ratio=SPHETModel.mg_ratio_eng_out  msk_plnt_m_r_ratio=SPHETModel.mg_ratio_mot_out  msk_plnt_s_r_ratio=1/SPHETModel.mg_ratio_out_gen  msk_plnt_s_c_ratio=1/SPHETModel.mg_ratio_eng_gen  msk_mtr_cont_trq=SPHETModel.cont_mtr_trq_map  msk_mtr_pk_trq=SPHETModel.peak_mtr_trq_map  msk_spd_bpt=SPHETModel.cont_mtr_trq_spdbpt  msk_gear_ratio=SPHETModel.mg_ratio_mot_out  msk_num_motors=1  msk_acc_trqmap=AccPdl_trqMap  msk_acc_spdbpt=AccPdl_spdbpt  msk_acc_pdlbpt=AccPdl_pdlbpt  msk_brk_trq=BrkPdl_brkTrq  msk_brk_pdlbpt=BrkPdl_pdlbpt
  Terminator : Terminator
  Unit Delay : UnitDelay  InitialCondition=3  SampleTime=-1
  Unit Delay1 : UnitDelay  InitialCondition=3  SampleTime=-1
  To_PCL : Outport
  wires:
  [gear_ratio] -> Bus Creator1/2  "gear_ratio"
  Series Parallel Hybrid Electric Truck Driver and Vehicle Acceleration Dynamics Model - Force Output/2 -> [gear_ratio]
  Series Parallel Hybrid Electric Powertrain Power Loss Model/1(PropSys_to_EMC) -> Series Parallel Hybrid Electric Post-Processing/1(PropSys_to_EMC), Series Parallel Hybrid Electric Truck Energy Management System/1(PropSys_to_EMC)
  Bus Selector2/1 -> 2 DOF Longitudinal Dynamics Model - Force Input/2  "<tail_grade_pct>"
  2 DOF Longitudinal Dynamics Model - Force Input/3 -> Bus Creator2/1  "F_prop"
  2 DOF Longitudinal Dynamics Model - Force Input/6 -> Bus Creator2/4  "F_rr"
  F_Dist_m/1 -> 2 DOF Longitudinal Dynamics Model - Force Input/3
  2 DOF Longitudinal Dynamics Model - Force Input/1 -> Bus Creator1/3, Series Parallel Hybrid Electric Truck Driver and Vehicle Acceleration Dynamics Model - Force Output/1  "vehSpdOut"
  Series Parallel Hybrid Electric Truck Driver and Vehicle Acceleration Dynamics Model - Force Output/3 -> 2 DOF Longitudinal Dynamics Model - Force Input/1  "F_cmd_out"
  Bus Creator2/1 -> Terminator/1
  2 DOF Longitudinal Dynamics Model - Force Input/7 -> Bus Creator3/1  "P_prop"
  2 DOF Longitudinal Dynamics Model - Force Input/10 -> Bus Creator3/4  "P_rr"
  2 DOF Longitudinal Dynamics Model - Force Input/8 -> Bus Creator3/2  "P_ar"
  Bus Creator1/1 -> Series Parallel Hybrid Electric Powertrain Power Loss Model/1(Motion_data_bus)  "MotionDatBus"
  2 DOF Longitudinal Dynamics Model - Force Input/2 -> Bus Creator1/4  "vehAccOut"
  V_SPD/1 -> Series Parallel Hybrid Electric Truck Driver and Vehicle Acceleration Dynamics Model - Force Output/3
  2 DOF Longitudinal Dynamics Model - Force Input/5 -> Bus Creator2/3  "F_cr"
  From_DTIL_BUS/1 -> Bus Selector3/1, Bus Selector2/1
  2 DOF Longitudinal Dynamics Model - Force Input/9 -> Bus Creator3/3  "P_cr"
  Bus Selector3/1 -> Series Parallel Hybrid Electric Powertrain Power Loss Model/3(clock)  "<clock>"
  Bus Creator3/1 -> Series Parallel Hybrid Electric Powertrain Power Loss Model/2(Power_data_bus)  "PowerDatBus"
  Series Parallel Hybrid Electric Post-Processing/1(To_PCL_BUS) -> Bus Selector1/1, To_PCL/1
  2 DOF Longitudinal Dynamics Model - Force Input/4 -> Bus Creator2/2  "F_ar"
  From_PCL/1 -> Bus Creator/3
  Series Parallel Hybrid Electric Truck Energy Management System/1(EMC_to_PropSys) -> Bus Selector/1, Series Parallel Hybrid Electric Powertrain Power Loss Model/4(EM_control_bus)
  Series Parallel Hybrid Electric Truck Driver and Vehicle Acceleration Dynamics Model - Force Output/1 -> [gear_cmd]
  [gear_cmd] -> Bus Creator1/1  "gear_cmd"
  Bus Selector/1 -> Series Parallel Hybrid Electric Truck Driver and Vehicle Acceleration Dynamics Model - Force Output/2  "<opt_gear>"
  Init_Pos_m/1 -> Series Parallel Hybrid Electric Powertrain Power Loss Model/5(Init_pos_m)
  Cd/1 -> 2 DOF Longitudinal Dynamics Model - Force Input/4
  Bus Creator/1 -> Series Parallel Hybrid Electric Truck Energy Management System/2(From_PCL_BUS)
  Bus Selector1/1 -> Unit Delay/1  "<blndElecEC_Wh_m>"
  Unit Delay/1 -> Bus Creator/1  "EC_Wh_m"
  Bus Selector1/2 -> Unit Delay1/1  "<DistTrvld_m>"
  Unit Delay1/1 -> Bus Creator/2  "DistTrvld_m"

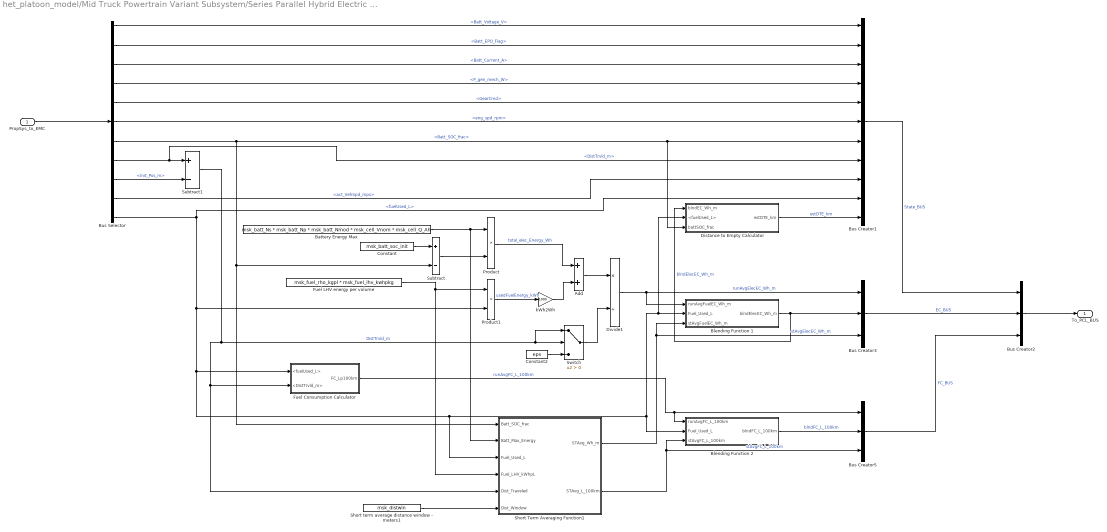
== system het_platoon_model/Mid Truck Powertrain Variant Subsystem/Series Parallel Hybrid Electric Truck/Series Parallel Hybrid Electric Post-Processing ==
  PropSys_to_EMC : Inport
  Add : Sum
  Battery Energy Max : Constant  Value=msk_batt_Ns * msk_batt_Np * msk_batt_Nmod * msk_cell_Vnom * msk_cell_Q_Ah
  Blending Function 1 : Subsystem
  Blending Function 2 : Subsystem
  Bus Creator1 : BusCreator  Inputs=11
  Bus Creator2 : BusCreator  Inputs=3
  Bus Creator3 : BusCreator  Inputs=3
  Bus Creator5 : BusCreator  Inputs=3
  Bus Selector : BusSelector  OutputSignals=Batt_Voltage_V,Batt_EPO_Flag,Batt_Current_A,P_gen_mech_W,GearCmd,eng_spd_rpm,Batt_SOC_frac,DistTrvld_m,Init_Pos_m,act_VehSpd_mps,fuelUsed_L
  Constant : Constant  Value=msk_batt_soc_init
  Constant2 : Constant  Value=eps
  Distance to Empty Calculator : Subsystem
  Divide1 : Product  Inputs=*/
  Fuel Consumption Calculator : Subsystem
  Fuel LHV energy per volume : Constant  Value=msk_fuel_rho_kgpl * msk_fuel_lhv_kwhpkg
  Product : Product
  Product1 : Product
  Short Term Averaging Function1 : MATLAB Function  TreatAsAtomicUnit=on
  Short term average distance window - meters1 : Constant  Value=msk_distwin
  Subtract : Sum  Inputs=+-
  Subtract1 : Sum  Inputs=+-
  Switch : Switch  Criteria=u2 > Threshold
  kWh2Wh : Gain  Gain=1000
  To_PCL_BUS : Outport
  wires:
  Add/1 -> Divide1/1
  Bus Selector/11 -> Bus Creator1/10, Fuel Consumption Calculator/1(<fuelUsed_L>), Short Term Averaging Function1/3(Fuel_Used_L), Blending Function 2/2(Fuel_Used_L), Blending Function 1/2(Fuel_Used_L), Distance to Empty Calculator/2(<fuelUsed_L>), Product1/2  "<fuelUsed_L>"
  Fuel Consumption Calculator/1(FC_Lp100km) -> Blending Function 2/1(runAvgFC_L_100km), Bus Creator5/1  "runAvgFC_L_100km"
  Fuel LHV energy per volume/1 -> Product1/1, Short Term Averaging Function1/4(Fuel_LHV_kWhpL)
  Short Term Averaging Function1/2(STAvg_L_100km) -> Blending Function 2/3(stAvgFC_L_100km), Bus Creator5/3  "stAvgFC_L_100km"
  Subtract1/1 -> Short Term Averaging Function1/5(Dist_Traveled), Fuel Consumption Calculator/2(<DistTrvld_m>), Switch/1, Switch/2  "DistTrvld_m"
  kWh2Wh/1 -> Add/2
  Blending Function 1/1(blndElecEC_Wh_m) -> Distance to Empty Calculator/1(blndEC_Wh_m), Bus Creator3/2  "blndElecEC_Wh_m"
  Short term average distance window - meters1/1 -> Short Term Averaging Function1/6(Dist_Window)
  Bus Creator3/1 -> Bus Creator2/2  "EC_BUS"
  Short Term Averaging Function1/1(STAvg_Wh_m) -> Bus Creator3/3, Blending Function 1/3(stAvgFuelEC_Wh_m)  "stAvgElecEC_Wh_m"
  Bus Selector/10 -> Bus Creator1/9  "<act_VehSpd_mps>"
  Divide1/1 -> Bus Creator3/1, Blending Function 1/1(runAvgFuelEC_Wh_m)  "runAvgElecEC_Wh_m"
  Blending Function 2/1(blndFC_L_100km) -> Bus Creator5/2  "blndFC_L_100km"
  Product1/1 -> kWh2Wh/1  "usedFuelEnergy_kWh"
  Bus Creator5/1 -> Bus Creator2/3  "FC_BUS"
  Bus Creator2/1 -> To_PCL_BUS/1
  Bus Creator1/1 -> Bus Creator2/1  "State_BUS"
  Battery Energy Max/1 -> Product/1, Short Term Averaging Function1/2(Batt_Max_Energy)
  Product/1 -> Add/1  "total_elec_Energy_Wh"
  Subtract/1 -> Product/2
  Constant/1 -> Subtract/1
  Bus Selector/7 -> Subtract/2, Short Term Averaging Function1/1(Batt_SOC_frac), Distance to Empty Calculator/3(battSOC_frac), Bus Creator1/7  "<Batt_SOC_frac>"
  PropSys_to_EMC/1 -> Bus Selector/1
  Switch/1 -> Divide1/2
  Constant2/1 -> Switch/3
  Distance to Empty Calculator/1(estDTE_km) -> Bus Creator1/11  "estDTE_km"
  Bus Selector/1 -> Bus Creator1/1  "<Batt_Voltage_V>"
  Bus Selector/2 -> Bus Creator1/2  "<Batt_EPO_Flag>"
  Bus Selector/3 -> Bus Creator1/3  "<Batt_Current_A>"
  Bus Selector/4 -> Bus Creator1/4  "<P_gen_mech_W>"
  Bus Selector/5 -> Bus Creator1/5  "<GearCmd>"
  Bus Selector/6 -> Bus Creator1/6  "<eng_spd_rpm>"
  Bus Selector/9 -> Subtract1/2  "<Init_Pos_m>"
  Bus Selector/8 -> Bus Creator1/8, Subtract1/1  "<DistTrvld_m>"
